simulink model "doc_pnseq2"  (Simulink 8.8)
settings: Solver=FixedStepDiscrete  StartTime=0.0  StopTime=93  RelTol=1e-3
PreLoadFcn:
  | iniStates = [ 0 0 1 0 1 1];
CloseFcn:
  | rtwprivate ssgencode ModelCloseRequest test1
settings Model: Creator=The MathWorks, Inc.  LastModifiedBy=acer
settings DataIOCC: SignalLoggingSaveFormat=Dataset
settings OptimizationCC: ExpressionDepthLimit=2147483647  InitFltsAndDblsToZero=on  LifeSpan=1
settings DebuggingCC: SaveWithParameterizedLinksMsg=none  SignalResolutionControl=TryResolveAllWithWarning  SolverPrmCheckMsg=warning  MultiTaskDSMMsg=warning  MultiTaskCondExecSysMsg=none  AllowSymbolicDim=off
settings RTWCC: SystemTargetFile=ert.tlc  GenCodeOnly=on  TemplateMakefile=ert_default_tmf  Description=Real-Time Workshop Embedded Coder (no auto configuration)
settings CodeAppCC: IgnoreCustomStorageClasses=off  CustomSymbolStrType=$N$R$M  InternalIdentifier=Classic
settings ERTTargetCC: TargetFcnLib=ansi_tfl_tmw.mat  MultiwordLength=2048  GenerateSampleERTMain=on  ERTCustomFileTemplate=example_file_process.tlc  ConvertIfToSwitch=off  SuppressUnreachableDefaultCases=off

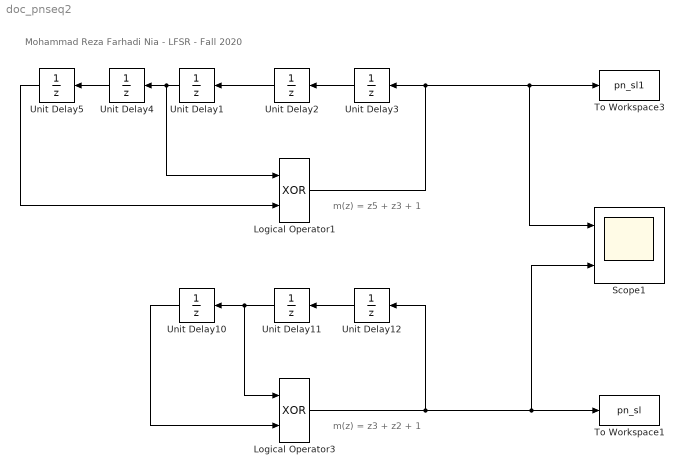
== system doc_pnseq2 ==
  note: Mohammad Reza Farhadi Nia - LFSR - Fall 2020
  note: m(z) = z3 + z2 + 1
  note: m(z) = z5 + z3 + 1
  Logical Operator1 : Logic  Operator=XOR  AllPortsSameDT=off  OutDataTypeStr=boolean
  Logical Operator3 : Logic  Operator=XOR  AllPortsSameDT=off  OutDataTypeStr=boolean
  Scope1 : Scope  NumInputPorts=2
      settings: Tag=1
  To Workspace1 : ToWorkspace  VariableName=pn_sl  SampleTime=-1
      settings: Save2DSignal=2-D array (concatenate along first dimension)
  To Workspace3 : ToWorkspace  VariableName=pn_sl1  SampleTime=-1
      settings: Save2DSignal=2-D array (concatenate along first dimension)
  Unit Delay{1,4..5,10} (4 alike) : UnitDelay  InitialCondition=iniStates(3)  SampleTime=-1
  Unit Delay11 : UnitDelay  InitialCondition=iniStates(2)  SampleTime=-1
  Unit Delay12 : UnitDelay  InitialCondition=iniStates(1)  SampleTime=-1
  Unit Delay2 : UnitDelay  InitialCondition=iniStates(2)  SampleTime=-1
  Unit Delay3 : UnitDelay  InitialCondition=iniStates(1)  SampleTime=-1
  wires:
  Unit Delay11/1 -> Logical Operator3/1, Unit Delay10/1
  Unit Delay12/1 -> Unit Delay11/1
  Unit Delay10/1 -> Logical Operator3/2
  Logical Operator1/1 -> Unit Delay3/1, Scope1/1, To Workspace3/1
  Unit Delay2/1 -> Unit Delay1/1
  Unit Delay3/1 -> Unit Delay2/1
  Unit Delay1/1 -> Logical Operator1/1, Unit Delay4/1
  Unit Delay4/1 -> Unit Delay5/1
  Unit Delay5/1 -> Logical Operator1/2
  Logical Operator3/1 -> Unit Delay12/1, To Workspace1/1, Scope1/2
